simulink model "vx_estimator_base"  (R2024b)
settings: Solver=VariableStepAuto  StartTime=0.0  StopTime=10.0  FixedStep=0.004  RelTol=1e-3
model workspace (MAT data in the model file):
  mbd_rack_movement = [-24.295 -24.2949831878 -24.2949831878 -24.2949831878 -24.2949831877 -24.2949831876 -24.2949831874 -24.2949831869 -24.2949831849 -24.2949831786 -24.2949831545 -24.2949831492 ... (273 elements, 273x1)]
  rack_mm = [-25.136 -25.1276327886 -25.1095284284 -25.0914240682 -25.073319708 -25.0564044471 -25.0415413809 -25.0266783147 -25.0118152486 -24.9987131808 -24.9886873592 -24.9786615375 ... (4070 elements, 4070x1)]
  steer_sensor = [701.530379071 702.453261845 703.675449618 704.897637391 706.119825165 707.135081137 707.617795373 708.10050961 708.583223846 709.091528196 709.761580489 710.431632781 ... (4070 elements, 4070x1)]
  wheel_steer_left = [22.9038666573 22.9079555 22.904490995 22.7859585761 22.785958576 22.7859585758 22.7859585755 22.7859585748 22.7859585724 22.7859585657 22.7859585412 22.7859585359 ... (273 elements, 273x1)]
  wheel_steer_right = [23.2682364009 23.2679586767 23.2681940775 23.3035254873 23.3035254873 23.3035254872 23.3035254871 23.3035254866 23.3035254847 23.3035254783 23.3035254538 23.3035254484 ... (273 elements, 273x1)]
libraries: matrix_library x2, simulink_extras x1, sharedTrackingLibrary x1
(part 1 of 2)
settings Model: Creator=ben  LastModifiedBy=lukec
settings OptimizationCC: DefaultParameterBehavior=Inlined  EnhancedBackFolding=on  PassReuseOutputArgsAs=Individual arguments  ZeroExternalMemoryAtStartup=off  ZeroInternalMemoryAtStartup=off  OptimizeBlockOrder=speed  DifferentSizesBufferReuse=on  OptimizationCustomize=off  EfficientTunableParamExpr=on
settings DebuggingCC: ParameterTunabilityLossMsg=error
settings HardwareCC: ProdBitPerPointer=32  ProdBitPerSizeT=32  ProdBitPerPtrDiffT=32  ProdLargestAtomicInteger=Long  ProdLargestAtomicFloat=Double  ProdWordSize=32  ProdHWDeviceType=ARM Compatible->ARM Cortex-M
settings SFSimCC: MATLABDynamicMemAlloc=off
settings RTWCC: Description=Embedded Coder  SystemTargetFile=ert.tlc  GenCodeOnly=on  PackageGeneratedCodeAndArtifacts=on  TemplateMakefile=ert_default_tmf  Toolchain=CMake  TargetLang=C++  HalideCodeGeneration=on
settings CodeAppCC: ForceParamTrailComments=on  IgnoreCustomStorageClasses=off  MaxIdLength=255  OperatorAnnotations=on  SimulinkDataObjDesc=on  SFDataObjDesc=on  InsertBlockDesc=on
settings ERTTargetCC: TargetLangStandard=C++17 (ISO)  CodeInterfacePackaging=C++ class  RootIOFormat=Structure reference  ERTCustomFileTemplate=example_file_process.tlc  ArrayContainerType=std::array

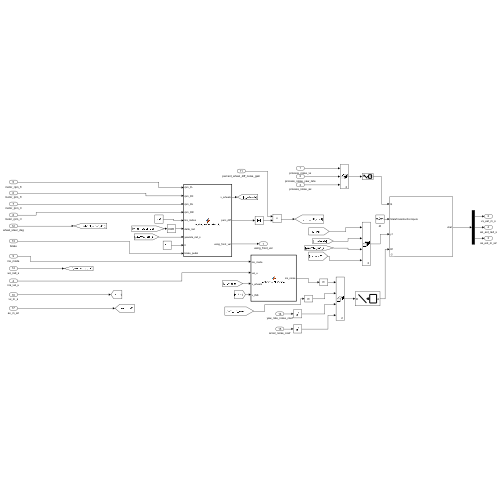
[thumbnail: Simulink's stored preview of the top-level diagram]
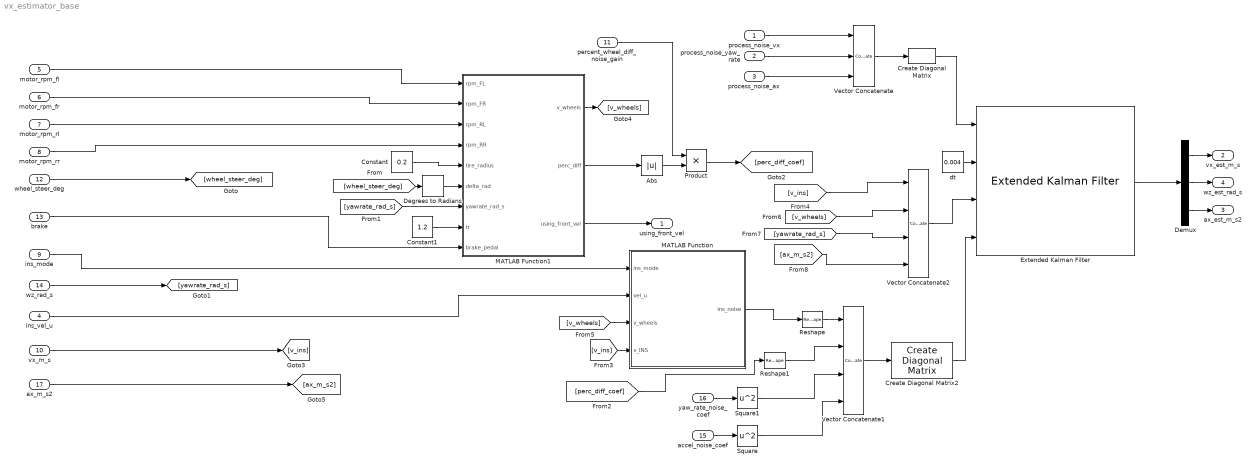
== system vx_estimator_base ==
  process_noise_vx : Inport  PortDimensions=1
  process_noise_yaw_rate : Inport  Port=2  PortDimensions=1
  process_noise_ax : Inport  Port=3  PortDimensions=1
  ins_vel_u : Inport  Port=4
  motor_rpm_fl : Inport  Port=5  PortDimensions=1
  motor_rpm_fr : Inport  Port=6  PortDimensions=1
  motor_rpm_rl : Inport  Port=7  PortDimensions=1
  motor_rpm_rr : Inport  Port=8  PortDimensions=1
  ins_mode : Inport  Port=9
  vx_m_s : Inport  Port=10  PortDimensions=1
  percent_wheel_diff_noise_gain : Inport  Port=11  PortDimensions=1
  wheel_steer_deg : Inport  Port=12  PortDimensions=1
  brake : Inport  Port=13  PortDimensions=1
  wz_rad_s : Inport  Port=14  PortDimensions=1
  accel_noise_coef : Inport  Port=15  PortDimensions=1
  yaw_rate_noise_coef : Inport  Port=16  PortDimensions=1
  ax_m_s2 : Inport  Port=17  PortDimensions=1
  Abs : Abs  SaturateOnIntegerOverflow=off
  Constant : Constant  Value=0.2
  Constant1 : Constant  Value=1.2
  Create Diagonal Matrix : matrix_library/Create Diagonal Matrix
      settings: LibrarySourceBlock=|
      | simulink/Matrix
      | Operations/Create Diagonal
      | Matrix
  Create Diagonal Matrix2 : matrix_library/Create Diagonal Matrix
      settings: LibrarySourceBlock=|
      | simulink/Matrix
      | Operations/Create Diagonal
      | Matrix
  Degrees to Radians : simulink_extras/Transformations/Degrees to Radians
  Demux : Demux  Outputs=3
  Extended Kalman Filter : sharedTrackingLibrary/Extended Kalman Filter  StateTransitionFcn=stateTransition  HasStateTransitionJacobianFcn=off  HasAdditiveProcessNoise=Additive  ProcessNoise=1  HasTimeVaryingProcessNoise=on  HasStateTransitionFcnExtraArgument=1  InitialState=[0;0;0]  InitialStateCovariance=[1;1;1]  MeasurementFcn1=measFunc  HasMeasurementJacobianFcn1=off  HasMeasurementEnablePort1=off  HasAdditiveMeasurementNoise1=Additive  MeasurementNoise1=1  HasTimeVaryingMeasurementNoise1=on  HasMeasurementFcnExtraArgument1=0  HasMeasurementWrapping1=off  MeasurementFcn2=myMeasurementFcn  HasMeasurementJacobianFcn2=off  HasMeasurementEnablePort2=off  HasAdditiveMeasurementNoise2=Additive  MeasurementNoise2=1  HasTimeVaryingMeasurementNoise2=off  HasMeasurementFcnExtraArgument2=0  HasMeasurementWrapping2=off  MeasurementFcn3=myMeasurementFcn  HasMeasurementJacobianFcn3=off  HasMeasurementEnablePort3=off  HasAdditiveMeasurementNoise3=Additive  MeasurementNoise3=1  HasTimeVaryingMeasurementNoise3=off  HasMeasurementFcnExtraArgument3=0  HasMeasurementWrapping3=off  MeasurementFcn4=myMeasurementFcn  HasMeasurementJacobianFcn4=off  HasMeasurementEnablePort4=off  HasAdditiveMeasurementNoise4=Additive  MeasurementNoise4=1  HasTimeVaryingMeasurementNoise4=off  HasMeasurementFcnExtraArgument4=0  HasMeasurementWrapping4=off  MeasurementFcn5=myMeasurementFcn  HasMeasurementJacobianFcn5=off  HasMeasurementEnablePort5=off  HasAdditiveMeasurementNoise5=Additive  MeasurementNoise5=1  HasTimeVaryingMeasurementNoise5=off  HasMeasurementFcnExtraArgument5=0  HasMeasurementWrapping5=off  EnableMultirate=off  StateTransitionFcnSampleTime=1  MeasurementFcn1SampleTime=1  MeasurementFcn2SampleTime=1  MeasurementFcn3SampleTime=1  MeasurementFcn4SampleTime=1  MeasurementFcn5SampleTime=1  UseCurrentEstimator=on  OutputStateCovariance=off  DataType=double  SampleTime=0.004  NumberOfMeasurements=1
  MATLAB Function : MATLAB Function  TreatAsAtomicUnit=on
  MATLAB Function1 : MATLAB Function  TreatAsAtomicUnit=on
  Product : Product
  Reshape : Reshape  OutputDimensionality=Customize
  Reshape1 : Reshape  OutputDimensionality=Customize
  Square : Math  Operator=square
  Square1 : Math  Operator=square
  Vector Concatenate : Concatenate  NumInputs=3  Mode=Multidimensional array  ConcatenateDimension=2
  Vector Concatenate1 : Concatenate  NumInputs=4  Mode=Multidimensional array  ConcatenateDimension=2
  Vector Concatenate2 : Concatenate  NumInputs=4  Mode=Multidimensional array  ConcatenateDimension=2
  dt : Constant  Value=0.004
  using_front_vel : Outport
  vx_est_m_s : Outport  Port=2
  ax_est_m_s2 : Outport  Port=3
  wz_est_rad_s : Outport  Port=4
  wires:
  Product/1 -> [perc_diff_coef]
  MATLAB Function1/1(v_wheels) -> [v_wheels]
  Demux/1 -> vx_est_m_s/1
  yaw_rate_noise_coef/1 -> Square1/1
  dt/1 -> Extended Kalman Filter/2
  Constant1/1 -> MATLAB Function1/8(tr)
  percent_wheel_diff_noise_gain/1 -> Product/1
  [wheel_steer_deg] -> Degrees to Radians/1
  [v_wheels] -> MATLAB Function/3(v_wheels)
  Vector Concatenate/1 -> Create Diagonal Matrix/1
  process_noise_vx/1 -> Vector Concatenate/1
  [yawrate_rad_s] -> Vector Concatenate2/3
  MATLAB Function1/2(perc_diff) -> Abs/1
  Extended Kalman Filter/1 -> Demux/1
  process_noise_ax/1 -> Vector Concatenate/3
  MATLAB Function1/3(using_front_vel) -> using_front_vel/1
  [yawrate_rad_s] -> MATLAB Function1/7(yawrate_rad_s)
  [perc_diff_coef] -> Reshape1/1
  [ax_m_s2] -> Vector Concatenate2/4
  [v_ins] -> Vector Concatenate2/1
  Degrees to Radians/1 -> MATLAB Function1/6(delta_rad)
  Square/1 -> Vector Concatenate1/4
  Vector Concatenate1/1 -> Create Diagonal Matrix2/1
  Square1/1 -> Vector Concatenate1/3
  [v_wheels] -> Vector Concatenate2/2
  Demux/2 -> wz_est_rad_s/1
  [v_ins] -> MATLAB Function/4(v_INS)
  Abs/1 -> Product/2
  Constant/1 -> MATLAB Function1/5(tire_radius)
  Create Diagonal Matrix2/1 -> Extended Kalman Filter/4
  Create Diagonal Matrix/1 -> Extended Kalman Filter/1
  process_noise_yaw_rate/1 -> Vector Concatenate/2
  accel_noise_coef/1 -> Square/1
  Demux/3 -> ax_est_m_s2/1
  Vector Concatenate2/1 -> Extended Kalman Filter/3
  MATLAB Function/1(ins_noise) -> Reshape/1
  Reshape/1 -> Vector Concatenate1/1
  Reshape1/1 -> Vector Concatenate1/2
  motor_rpm_fl/1 -> MATLAB Function1/1(rpm_FL)
  motor_rpm_fr/1 -> MATLAB Function1/2(rpm_FR)
  motor_rpm_rl/1 -> MATLAB Function1/3(rpm_RL)
  motor_rpm_rr/1 -> MATLAB Function1/4(rpm_RR)
  wheel_steer_deg/1 -> [wheel_steer_deg]
  brake/1 -> MATLAB Function1/9(brake_pedal)
  ins_mode/1 -> MATLAB Function/1(ins_mode)
  wz_rad_s/1 -> [yawrate_rad_s]
  ins_vel_u/1 -> MATLAB Function/2(vel_u)
  vx_m_s/1 -> [v_ins]
  ax_m_s2/1 -> [ax_m_s2]
